simulink model "washout_prototype"  (R2020a)
settings: Solver=FixedStepDiscrete  StartTime=0.0  StopTime=inf  FixedStep=0.002  RelTol=1e-3  EnableMultiTasking=on
values from neighbouring files (symbols this model uses):
  reg_k = 0.5    [washout_filter_design.m]
libraries: cstblocks x1
settings Model: ExtModeTrigDuration=10000  Creator=vinja  LastModifiedBy=vinja
settings SolverCC: PositivePriorityOrder=on
settings DataIOCC: ReturnWorkspaceOutputs=off
settings OptimizationCC: LifeSpan=inf
settings DebuggingCC: ArithmeticOperatorsInVariantConditions=warning
settings SFSimCC: SimUseLocalCustomCode=off  CustomCodeUndefinedFunction=UseInterfaceOnly
settings RTWCC: Description=QUARC Win64 Target  SystemTargetFile=quarc_win64.tlc  TemplateMakefile=quarc_default_tmf  RTWUseLocalCustomCode=off
settings CodeAppCC: StateflowObjectComments=on
settings STFCustomTargetCC: TargetPreCompLibLocation=C:\PROGRA~3\QUARC\lib\2016a\win64\release  TargetLangStandard=C99 (ISO)  ConcurrentExecutionCompliant=on  GRTInterface=on  SystemTargetFile=quarc_win64.tlc
settings GRTTargetCC: TargetPreCompLibLocation=C:\PROGRA~3\QUARC\lib\2016a\win64\release  ParMdlRefBuildCompliant=off  CompOptLevelCompliant=off  CombineOutputUpdateFcns=off  MatFileLogging=off  CPPClassGenCompliant=off  GRTInterface=on  UseToolchainInfoCompliant=off  ExtMode=on  ExtModeMexFile=quarc_comm
settings ConfigComp: CovMetricSettings=dswe

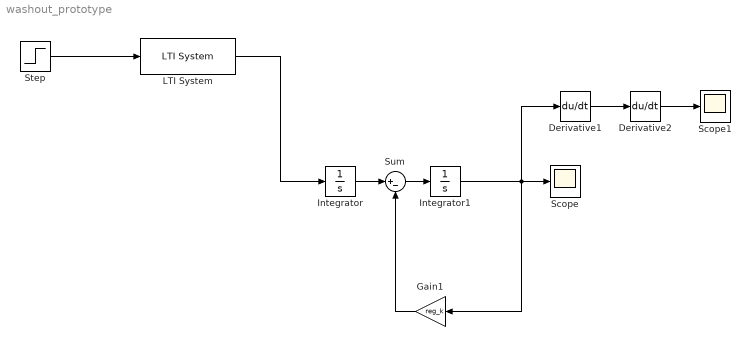
== system washout_prototype ==
  Derivative1 : Derivative
  Derivative2 : Derivative
  Gain1 : Gain  Gain=reg_k
  Integrator : Integrator
  Integrator1 : Integrator
  LTI System : cstblocks/LTI System  sys=g_hp  IC=[]
  Scope : Scope
  Scope1 : Scope
  Step : Step  After=2*9.81  SampleTime=0
  Sum : Sum  Inputs=|+-
  wires:
  LTI System/1 -> Integrator/1
  Derivative2/1 -> Scope1/1
  Sum/1 -> Integrator1/1
  Integrator/1 -> Sum/1
  Gain1/1 -> Sum/2
  Step/1 -> LTI System/1
  Integrator1/1 -> Derivative1/1, Gain1/1, Scope/1
  Derivative1/1 -> Derivative2/1
